simulink model "Data_acq"  (R2022b)
settings: Solver=VariableStepAuto  StartTime=0.0  StopTime=inf  RelTol=1e-3
values from neighbouring files (symbols this model uses):
  Kd = place(Ad,Bd,p_discretos)    [Sist_ident.m]
undefined symbols (not defined in the file or in its folder): daq
libraries: daqlib x2
settings Model: Creator=juand  LastModifiedBy=juand

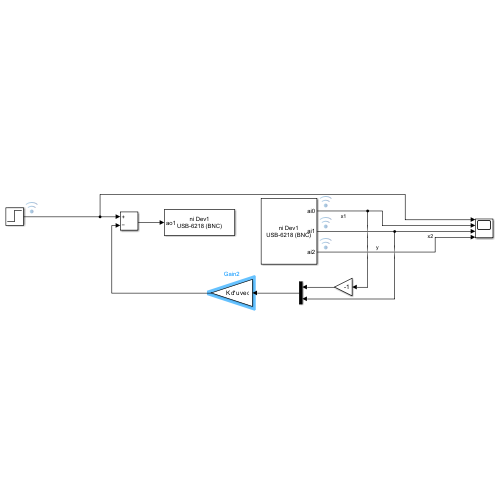
[thumbnail: Simulink's stored preview of the top-level diagram]
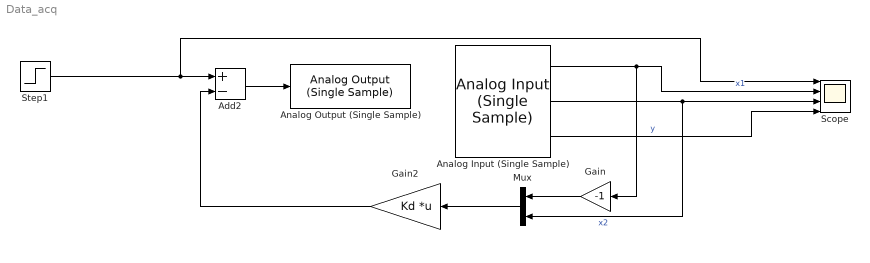
== system Data_acq ==
  Add2 : Sum  Inputs=+-
  Analog Input (Single Sample) : daqlib/Analog Input (Single Sample)  DeviceMenu=(none)  Device=ni Dev1 (USB-6218 (BNC))  ObjConstructor=daq.createSession('ni')  BlockSampleTime=0.048828  NChannelsSelected=3  Channels=1$ai0$$Dev1$1$4$3$1$#1$ai1$$Dev1$1$4$3$1$#1$ai2$$Dev1$1$4$3$1$#0$ai3$$Dev1$1$4$3$1$#0$ai4$$Dev1$1$4$3$1$#0$ai5$$Dev1$1$4$3$1$#0$ai6$$Dev1$1$4$3$1$#0$ai7$$Dev1$1$4$3$1$#0$ai8$$Dev1$1$4$1$1$#0$ai9$$Dev1$1$4$1$1$#0$ai10$$Dev1$1$4$1$1$#0$ai11$$Dev1$1$4$1$1$#0$ai12$$Dev1$1$4$1$1$#0$ai13$$Dev1$1$4$1$1$#0$ai14$$Dev1$1$4$1$1$#0$ai15$$Dev1$1$4$1$1$#0$ai16$$Dev1$1$4$3$1$#0$ai17$$Dev1$1$4$3$1$#0$ai18$$Dev1$1$4$3$1$#0$ai19$$Dev1$1$4$3$1$#0$ai20$$Dev1$1$4$3$1$#0$ai21$$Dev1$1$4$3$1$#0$ai22$$Dev1$1$4$3$1$#0$ai23$$Dev1$1$4$3$1$#0$ai24$$Dev1$1$4$1$1$#0$ai25$$Dev1$1$4$1$1$#0$ai26$$Dev1$1$4$1$1$#0$ai27$$Dev1$1$4$1$1$#0$ai28$$Dev1$1$4$1$1$#0$ai29$$Dev1$1$4$1$1$#0$ai30$$Dev1$1$4$1$1$#0$ai31$$Dev1$1$4$1$1$#  NPorts=1 per channel  OutputTimestamp=off
  Analog Output (Single Sample) : daqlib/Analog Output (Single Sample)  DeviceMenu=(none)  Device=ni Dev1 (USB-6218 (BNC))  ObjConstructor=daq.createSession('ni')  NChannelsSelected=1  Channels=0$ao0$$Dev1$1$1$N/A$#1$ao1$$Dev1$1$1$N/A$#  NPorts=1 per channel  BlockSampleTime=0.048828
  Gain : Gain  Gain=-1
  Gain2 : Gain  Gain=Kd  Multiplication=Matrix(K*u) (u vector)
  Mux : Mux  Inputs=2
  Scope : Scope  NumInputPorts=4
  Step1 : Step  After=1/0.51  SampleTime=0.048828
  wires:
  Mux/1 -> Gain2/1
  Gain2/1 -> Add2/2
  Gain/1 -> Mux/1
  Add2/1 -> Analog Output (Single Sample)/1
  Analog Input (Single Sample)/1 -> Gain/1, Scope/2  "x1"
  Analog Input (Single Sample)/2 -> Mux/2, Scope/3  "x2"
  Analog Input (Single Sample)/3 -> Scope/4  "y"
  Step1/1 -> Scope/1, Add2/1
